simulink model "ammclib_amclib_observer_FLT_s32k14x"  (Simulink 9.0)
settings: Solver=FixedStepDiscrete  StartTime=0.0  StopTime=10  FixedStep=0.001  RelTol=1e-3  EnableMultiTasking=on
PostLoadFcn:
  | ammclib_amclib_observer_s32k14x_param();
InitFcn:
  | mbd_s32k_consistency_checks(bdroot(gcs));
undefined symbols (not defined in the file or in its folder): LQFP
libraries: ammclib_bam_s32k14x x18, mbd_s32k1xx_ec_toolbox x2, simulink x1
Description:
  | This model tests the AMMCLIB AMCLIB OBSERVER FLT blocks
  | 
  | Validation:
  | - Run the model in Simulation and check the results
  | - Open Freemaster (ammclib_amclib_observer_FLT_s32k14x.pmp) and compare the HW results against the Simulated ones
CloseFcn:
  | clear all;
settings Model: Creator=NXP MBDT Team  LastModifiedBy=nxf35172
settings DataIOCC: ExternalInput=off  InitialState=off  LimitDataPoints=on  SaveOutput=off  SignalLogging=off  SaveTime=off
settings OptimizationCC: DefaultParameterBehavior=Inlined  LifeSpan=1
settings DebuggingCC: SolverPrmCheckMsg=warning  InheritedTsInSrcMsg=none  SingleTaskRateTransMsg=error  IntegerOverflowMsg=none  ParameterPrecisionLossMsg=none  UnconnectedInputMsg=error  UnconnectedOutputMsg=error  UnconnectedLineMsg=error  AllowSymbolicDim=off  UnknownTsInhSupMsg=error  StateNameClashWarn=warning
settings HardwareCC: ProdLargestAtomicInteger=Long  ProdLargestAtomicFloat=Double  ProdEndianess=LittleEndian  ProdHWDeviceType=ARM Compatible->ARM Cortex
settings SFSimCC: MATLABDynamicMemAlloc=off
settings RTWCC: SystemTargetFile=mbd_s32k.tlc  MakeCommand=mbd_s32k_make_rtw COPY_MDLREF_INCLUDES=0  TemplateMakefile=mbd_s32k.tmf  Description=Model Based Design Toolbox S32K14x Code Generation Target
settings CodeAppCC: IgnoreCustomStorageClasses=off
settings STFCustomTargetCC: CombineOutputUpdateFcns=on  ERTCustomFileBanners=on  SupportContinuousTime=off  SupportNonInlinedSFcns=off  RemoveResetFunc=on  MATLABClassNameForMDSCustomization=Simulink.SoftwareTarget.ERTCustomization  GRTInterface=off  SystemTargetFile=mbd_s32k14.tlc
settings ERTTargetCC: MultiwordLength=2048  ParMdlRefBuildCompliant=off  CompOptLevelCompliant=off  ConcurrentExecutionCompliant=off  ModelStepFunctionPrototypeControlCompliant=off  CPPClassGenCompliant=off  UseToolchainInfoCompliant=off  InlinedParameterPlacement=NonHierarchical  ERTCustomFileTemplate=example_file_process.tlc  ConvertIfToSwitch=off  SuppressUnreachableDefaultCases=off

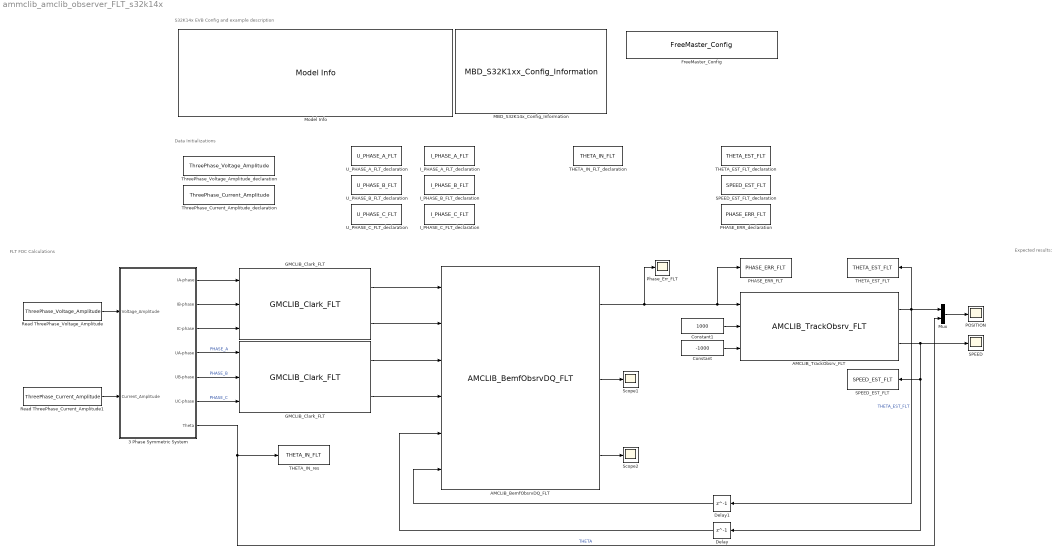
== system ammclib_amclib_observer_FLT_s32k14x ==
  note: Expected results:
  note: S32K14x EVB Config and example description
  note: Data Initializations
  note: FLT FOC Calculations
  " Read ThreePhase_Current_Amplitude1" : DataStoreRead  DataStoreName=ThreePhase_Current_Amplitude
  " Read ThreePhase_Voltage_Amplitude" : DataStoreRead  DataStoreName=ThreePhase_Voltage_Amplitude
  3 Phase Symmetric System : Subsystem
  AMCLIB_BemfObsrvDQ_FLT : ammclib_bam_s32k14x/AMCLIB/bam_flt/AMCLIB_BemfObsrvDQ_FLT  fltIGain=fltIGain  fltUGain=fltUGain  fltWIGain=fltWIGain  fltEGain=fltEGain  fltCC1sc_D=fltCC1sc_D  fltCC1sc_Q=fltCC1sc_Q  fltCC2sc_D=fltCC2sc_D  fltCC2sc_Q=fltCC2sc_Q  fltUpperLimit_D=fltUpperLimit_D  fltUpperLimit_Q=fltUpperLimit_Q  fltLowerLimit_D=fltLowerLimit_D  fltLowerLimit_Q=fltLowerLimit_Q
  AMCLIB_TrackObsrv_FLT : ammclib_bam_s32k14x/AMCLIB/bam_flt/AMCLIB_TrackObsrv_FLT  fltCC1=fltCC1  fltCC2=fltCC2  fltC1=fltC1
  Constant : Constant  Value=-1000  OutDataTypeStr=Inherit: Inherit via back propagation
  Constant1 : Constant  Value=1000  OutDataTypeStr=Inherit: Inherit via back propagation
  Delay : Delay  DelayLength=1  InitialCondition=0
  Delay1 : Delay  DelayLength=1  InitialCondition=0
  FreeMaster_Config : mbd_s32k1xx_ec_toolbox/Utility Blocks/FreeMaster_Config  interface=LPUART1  baudrate=115200  rxd=PTC6: [LPUART1_RX | Receive]  txd=PTC7: [LPUART1_TX | Transmit]  mode=Short Interrupt  isr_prio=1  show_adv_opts=on  use_scope=on  max_scope_vars=8  use_recorder=on  max_rec_vars=8  rec_buff_size=1024  rec_timebase=0 milliseconds  comm_buffer_size_auto=on  comm_buffer_size=255  comm_rqueue_size_default=on  comm_rqueue_size=32
  GMCLIB_Clark_FLT : ammclib_bam_s32k14x/GMCLIB/bam_flt/GMCLIB_Clark_FLT
  "GMCLIB_Clark_FLT " : ammclib_bam_s32k14x/GMCLIB/bam_flt/GMCLIB_Clark_FLT
  I_PHASE_A_FLT_declaration : DataStoreMemory  Priority=2  DataStoreName=I_PHASE_A_FLT  ReadBeforeWriteMsg=warning  WriteAfterWriteMsg=warning  WriteAfterReadMsg=warning  ShowAdditionalParam=off  OutDataTypeStr=single
  I_PHASE_B_FLT_declaration : DataStoreMemory  Priority=2  DataStoreName=I_PHASE_B_FLT  ReadBeforeWriteMsg=warning  WriteAfterWriteMsg=warning  WriteAfterReadMsg=warning  ShowAdditionalParam=off  OutDataTypeStr=single
  I_PHASE_C_FLT_declaration : DataStoreMemory  Priority=2  DataStoreName=I_PHASE_C_FLT  ReadBeforeWriteMsg=warning  WriteAfterWriteMsg=warning  WriteAfterReadMsg=warning  ShowAdditionalParam=off  OutDataTypeStr=single
  MBD_S32K14x_Config_Information : mbd_s32k1xx_ec_toolbox/MBD_S32K1xx_Config_Information  Priority=0  mbdt_ver=0  disp_str=|  config_params=[]  mcu_target_name=S32K144  mcu_target_package=100-LQFP  mcu_target_sram_size=64KB  mcu_system_clock_freq=80  mcu_xtal_freq=External 8  mcu_steptick_timer=LPIT Channel 0  mcu_steptick_prio=15  ds_import_enable=on  target_compiler=GCC  target_memory=FLASH  gcc_target_compile_opts=-mcpu=cortex-m4 -mthumb -mfloat-abi=hard -mfpu=fpv4-sp-d16 -O1 -g -gstrict-dwarf  gcc_target_assemble_opts=-mcpu=cortex-m4 -mthumb -mfloat-abi=hard -mfpu=fpv4-sp-d16 -g  gcc_target_link_opts=-mcpu=cortex-m4 -mthumb -mfloat-abi=hard -mfpu=fpv4-sp-d16  gcc_target_default_lcf=on  gcc_target_user_lcf=S32K144_64_flash.ld  ghs_target_compile_opts=-cpu=cortexm4f -thumb -DARM_MATH_CM4 -fpu=vfpv4_d16 -fsingle -Ogeneral -Wundef -Wimplicit-int -Wshadow -Wtrigraphs --no_commons --gnu_asm -gnu99 -gdwarf-2 -G  ghs_target_assemble_opts=-cpu=cortexm4f -fpu=vfpv4_d16  ghs_target_link_opts=-cpu=cortexm4f -thumb -fpu=vfpv4_d16  ghs_target_default_lcf=off  ghs_target_user_lcf=S32K144_64_flash.ld  iar_target_compile_opts=--cpu=Cortex-M4F --thumb --fpu=VFPv4_sp -Ol -e --debug --dlib_config normal  iar_target_assemble_opts=--cpu Cortex-M4F --thumb --fpu VFPv4_sp  iar_target_link_opts=--no_exceptions --vfe --inline  iar_target_default_lcf=off  iar_target_user_lcf=S32K144_64_flash.icf  pil_download_enable=off  rbl_download_enable=on  rbl_start_delay=5000000  rbl_download_interface=OpenSDA  rbl_restart_request=off  rbl_com_port=Custom  rbl_com_port_custom=COM1  pil_download_rate=57600  pil_opensda_drive=Custom  pil_opensda_drive_custom=D  pil_uart_instance=0  pil_uart_rx=PTA2: [LPUART0_RX | Receive]  pil_uart_tx=PTA3: [LPUART0_TX | Transmit]  FTM_PWM_PcrCheckEnDis=on  FTM_Input_Edge_Inputs_PcrCheckEnDis=on  FTM_Dual_Edge_Inputs_PcrCheckEnDis=on  FTM_Quadrature_Inputs_PcrCheckEnDis=on  FTM_Hall_Sensor_Inputs_PcrCheckEnDis=on  LPTMR_PcrCheckEnDis=on  PIT_PcrCheckEnDis=on  RTC_PcrCheckEnDis=on  FlexCAN_PcrCheckEnDis=on  LIN_PcrCheckEnDis=on  FlexIO_PcrCheckEnDis=on  LPI2C_PcrCheckEnDis=on  LPSPI_PcrCheckEnDis=on  LPUART_PcrCheckEnDis=on  CMP_PcrCheckEnDis=on  GPIO_OutputPcrCheckEnDis=on  GPIO_InputPcrCheckEnDis=on  SBC_PcrCheckEnDis=on  AMMCLIB_PcrCheckEnDis=on  FM_PcrCheckEnDis=on  Profile_PcrCheckEnDis=on  ConfigParams_PcrCheckEnDis=on  ModelRef_PcrCheckEnDis=on  PDB0_PcrCheckEnDis=on  CSEc_PcrCheckEnDis=on  eDMA_PcrCheckEnDis=on  ADC_PcrCheckEnDis=on  WDOG_PcrCheckEnDis=on
      | Target : S32K142-16KB_SRAM
      | Package : 100-pin
      | System clock : 80 MHz
      | XTAL clock : External 8 MHz
      | Compiler : GCC
      | Target Type : FLASH
      | Download Code after build : (OpenSDA: E)
      | Step Tick Interrupt Priority : 15
  Model Info : simulink/Model-Wide Utilities/Model Info  Frame=off  DisplayStringWithTags=|  HorizontalTextAlignment=Left  LeftAlignmentValue=0.02
      | Model Name: %<ModelName>
      | 
      | Description: %<Description>
  Mux : Mux  Inputs=2
  PHASE_ERR_FLT : DataStoreWrite  DataStoreName=PHASE_ERR_FLT
  PHASE_ERR_declaration : DataStoreMemory  Priority=2  DataStoreName=PHASE_ERR_FLT  ReadBeforeWriteMsg=warning  WriteAfterWriteMsg=warning  WriteAfterReadMsg=warning  ShowAdditionalParam=off  OutDataTypeStr=single
  POSITION : Scope
  Phase_Err_FLT : Scope
  SPEED : Scope
  SPEED_EST_FLT : DataStoreWrite  DataStoreName=SPEED_EST_FLT
  SPEED_EST_FLT_declaration : DataStoreMemory  Priority=2  DataStoreName=SPEED_EST_FLT  ReadBeforeWriteMsg=warning  WriteAfterWriteMsg=warning  WriteAfterReadMsg=warning  ShowAdditionalParam=off  OutDataTypeStr=single
  Scope1 : Scope
  Scope2 : Scope
  THETA_EST_FLT : DataStoreWrite  DataStoreName=THETA_EST_FLT
  THETA_EST_FLT_declaration : DataStoreMemory  Priority=2  DataStoreName=THETA_EST_FLT  ReadBeforeWriteMsg=warning  WriteAfterWriteMsg=warning  WriteAfterReadMsg=warning  ShowAdditionalParam=off  OutDataTypeStr=single
  THETA_IN_FLT_declaration : DataStoreMemory  Priority=2  DataStoreName=THETA_IN_FLT  ReadBeforeWriteMsg=warning  WriteAfterWriteMsg=warning  WriteAfterReadMsg=warning  ShowAdditionalParam=off  OutDataTypeStr=single
  THETA_IN_res : DataStoreWrite  DataStoreName=THETA_IN_FLT
  ThreePhase_Current_Amplitude_declaration : DataStoreMemory  Priority=1  DataStoreName=ThreePhase_Current_Amplitude  WriteAfterWriteMsg=warning  WriteAfterReadMsg=warning  InitialValue=0.3  ShowAdditionalParam=off  OutMin=-1  OutMax=1  OutDataTypeStr=single
  ThreePhase_Voltage_Amplitude_declaration : DataStoreMemory  Priority=1  DataStoreName=ThreePhase_Voltage_Amplitude  WriteAfterWriteMsg=warning  WriteAfterReadMsg=warning  InitialValue=0.61  ShowAdditionalParam=off  OutMin=-1  OutMax=1  OutDataTypeStr=single
  U_PHASE_A_FLT_declaration : DataStoreMemory  Priority=2  DataStoreName=U_PHASE_A_FLT  ReadBeforeWriteMsg=warning  WriteAfterWriteMsg=warning  WriteAfterReadMsg=warning  ShowAdditionalParam=off  OutDataTypeStr=single
  U_PHASE_B_FLT_declaration : DataStoreMemory  Priority=2  DataStoreName=U_PHASE_B_FLT  ReadBeforeWriteMsg=warning  WriteAfterWriteMsg=warning  WriteAfterReadMsg=warning  ShowAdditionalParam=off  OutDataTypeStr=single
  U_PHASE_C_FLT_declaration : DataStoreMemory  Priority=2  DataStoreName=U_PHASE_C_FLT  ReadBeforeWriteMsg=warning  WriteAfterWriteMsg=warning  WriteAfterReadMsg=warning  ShowAdditionalParam=off  OutDataTypeStr=single
  wires:
  3 Phase Symmetric System/7(Theta) -> Mux/2, THETA_IN_res/1  "THETA"
  " Read ThreePhase_Voltage_Amplitude"/1 -> 3 Phase Symmetric System/1("Voltage_Amplitude ")
  AMCLIB_BemfObsrvDQ_FLT/2 -> Scope1/1
  AMCLIB_BemfObsrvDQ_FLT/3 -> Scope2/1
  " Read ThreePhase_Current_Amplitude1"/1 -> 3 Phase Symmetric System/2(Current_Amplitude)
  GMCLIB_Clark_FLT/1 -> AMCLIB_BemfObsrvDQ_FLT/1
  GMCLIB_Clark_FLT/2 -> AMCLIB_BemfObsrvDQ_FLT/2
  "GMCLIB_Clark_FLT "/1 -> AMCLIB_BemfObsrvDQ_FLT/3
  "GMCLIB_Clark_FLT "/2 -> AMCLIB_BemfObsrvDQ_FLT/4
  3 Phase Symmetric System/1(IA-phase) -> GMCLIB_Clark_FLT/1
  3 Phase Symmetric System/2(IB-phase) -> GMCLIB_Clark_FLT/2
  3 Phase Symmetric System/3(IC-phase) -> GMCLIB_Clark_FLT/3
  3 Phase Symmetric System/4(UA-phase) -> "GMCLIB_Clark_FLT "/1  "PHASE_A"
  3 Phase Symmetric System/5(UB-phase) -> "GMCLIB_Clark_FLT "/2  "PHASE_B"
  3 Phase Symmetric System/6(UC-phase) -> "GMCLIB_Clark_FLT "/3  "PHASE_C"
  AMCLIB_BemfObsrvDQ_FLT/1 -> PHASE_ERR_FLT/1, AMCLIB_TrackObsrv_FLT/1, Phase_Err_FLT/1
  Constant/1 -> AMCLIB_TrackObsrv_FLT/3
  Constant1/1 -> AMCLIB_TrackObsrv_FLT/2
  AMCLIB_TrackObsrv_FLT/1 -> THETA_EST_FLT/1, Mux/1, Delay1/1  "THETA_EST_FLT"
  AMCLIB_TrackObsrv_FLT/2 -> SPEED_EST_FLT/1, Delay/1, SPEED/1
  Delay/1 -> AMCLIB_BemfObsrvDQ_FLT/5
  Delay1/1 -> AMCLIB_BemfObsrvDQ_FLT/6
  Mux/1 -> POSITION/1

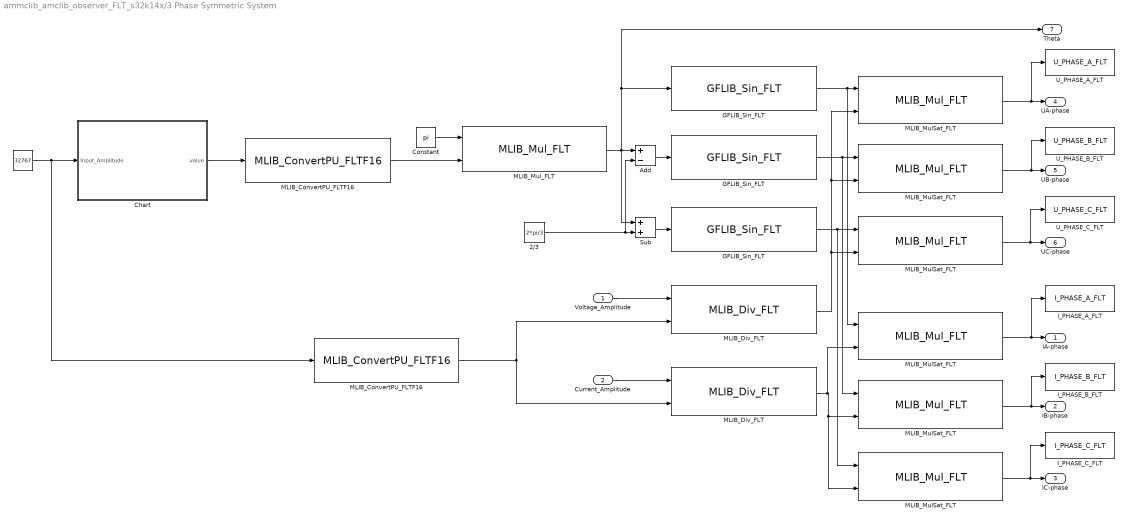
== system ammclib_amclib_observer_FLT_s32k14x/3 Phase Symmetric System ==
  "Voltage_Amplitude " : Inport
  Current_Amplitude : Inport  Port=2
  " " : Constant  Value=32767  OutDataTypeStr=int16
  2/3 : Constant  Value=2*pi/3  OutDataTypeStr=single
  Add : Sum  Inputs=+-
  Chart : Stateflow chart  TreatAsAtomicUnit=on
  Constant : Constant  Value=pi  OutDataTypeStr=Inherit: Inherit via back propagation
  GFLIB_Sin_FLT : ammclib_bam_s32k14x/GFLIB/bam_flt/GFLIB_Sin_FLT
  "GFLIB_Sin_FLT " : ammclib_bam_s32k14x/GFLIB/bam_flt/GFLIB_Sin_FLT
  "GFLIB_Sin_FLT  " : ammclib_bam_s32k14x/GFLIB/bam_flt/GFLIB_Sin_FLT
  I_PHASE_A_FLT : DataStoreWrite  DataStoreName=I_PHASE_A_FLT
  I_PHASE_B_FLT : DataStoreWrite  DataStoreName=I_PHASE_B_FLT
  I_PHASE_C_FLT : DataStoreWrite  DataStoreName=I_PHASE_C_FLT
  MLIB_ConvertPU_FLTF16 : ammclib_bam_s32k14x/MLIB/bam_flt/MLIB_ConvertPU_FLTF16
  "MLIB_ConvertPU_FLTF16    " : ammclib_bam_s32k14x/MLIB/bam_flt/MLIB_ConvertPU_FLTF16
  MLIB_Div_FLT : ammclib_bam_s32k14x/MLIB/bam_flt/MLIB_Div_FLT
  "MLIB_Div_FLT  " : ammclib_bam_s32k14x/MLIB/bam_flt/MLIB_Div_FLT
  MLIB_MulSat_FLT : ammclib_bam_s32k14x/MLIB/bam_flt/MLIB_Mul_FLT
  "MLIB_MulSat_FLT " : ammclib_bam_s32k14x/MLIB/bam_flt/MLIB_Mul_FLT
  "MLIB_MulSat_FLT  " : ammclib_bam_s32k14x/MLIB/bam_flt/MLIB_Mul_FLT
  "MLIB_MulSat_FLT   " : ammclib_bam_s32k14x/MLIB/bam_flt/MLIB_Mul_FLT
  "MLIB_MulSat_FLT    " : ammclib_bam_s32k14x/MLIB/bam_flt/MLIB_Mul_FLT
  "MLIB_MulSat_FLT     " : ammclib_bam_s32k14x/MLIB/bam_flt/MLIB_Mul_FLT
  MLIB_Mul_FLT : ammclib_bam_s32k14x/MLIB/bam_flt/MLIB_Mul_FLT
  Sub : Sum
  U_PHASE_A_FLT : DataStoreWrite  DataStoreName=U_PHASE_A_FLT
  U_PHASE_B_FLT : DataStoreWrite  DataStoreName=U_PHASE_B_FLT
  U_PHASE_C_FLT : DataStoreWrite  DataStoreName=U_PHASE_C_FLT
  IA-phase : Outport
  IB-phase : Outport  Port=2
  IC-phase : Outport  Port=3
  UA-phase : Outport  Port=4
  UB-phase : Outport  Port=5
  UC-phase : Outport  Port=6
  Theta : Outport  Port=7
  wires:
  2/3/1 -> Add/2, Sub/2
  Sub/1 -> "GFLIB_Sin_FLT  "/1
  Add/1 -> "GFLIB_Sin_FLT "/1
  "Voltage_Amplitude "/1 -> MLIB_Div_FLT/1
  MLIB_Div_FLT/1 -> "MLIB_MulSat_FLT  "/2, "MLIB_MulSat_FLT "/2, MLIB_MulSat_FLT/2
  GFLIB_Sin_FLT/1 -> "MLIB_MulSat_FLT   "/1, MLIB_MulSat_FLT/1
  "GFLIB_Sin_FLT "/1 -> "MLIB_MulSat_FLT    "/1, "MLIB_MulSat_FLT "/1
  "GFLIB_Sin_FLT  "/1 -> "MLIB_MulSat_FLT     "/1, "MLIB_MulSat_FLT  "/1
  "MLIB_MulSat_FLT "/1 -> U_PHASE_B_FLT/1, UB-phase/1
  "MLIB_MulSat_FLT  "/1 -> U_PHASE_C_FLT/1, UC-phase/1
  " "/1 -> Chart/1(Input_Amplitude), "MLIB_ConvertPU_FLTF16    "/1
  MLIB_MulSat_FLT/1 -> U_PHASE_A_FLT/1, UA-phase/1
  Current_Amplitude/1 -> "MLIB_Div_FLT  "/1
  "MLIB_MulSat_FLT    "/1 -> IB-phase/1, I_PHASE_B_FLT/1
  "MLIB_MulSat_FLT     "/1 -> IC-phase/1, I_PHASE_C_FLT/1
  "MLIB_MulSat_FLT   "/1 -> IA-phase/1, I_PHASE_A_FLT/1
  "MLIB_Div_FLT  "/1 -> "MLIB_MulSat_FLT   "/2, "MLIB_MulSat_FLT     "/2, "MLIB_MulSat_FLT    "/2
  MLIB_Mul_FLT/1 -> Theta/1, GFLIB_Sin_FLT/1, Sub/1, Add/1
  "MLIB_ConvertPU_FLTF16    "/1 -> MLIB_Div_FLT/2, "MLIB_Div_FLT  "/2
  MLIB_ConvertPU_FLTF16/1 -> MLIB_Mul_FLT/2
  Constant/1 -> MLIB_Mul_FLT/1
  Chart/1(value) -> MLIB_ConvertPU_FLTF16/1

== stateflow chart 3 Phase Symmetric System/Chart ==
  settings: executeAtInitialization=1
  state A
    du:
    cntr=cntr+25;
    value=cntr;
    ex:
    cntr = -Input_Amplitude;
  (default) -> A : {cntr=0;}
  A -> A : [cntr >= Input_Amplitude]
  data: cntr local int16 =0; value output int16; Input_Amplitude input int16
